simulink model "plant"  (R2016a)
settings: Solver=ode45  StartTime=0.0  StopTime=12  RelTol=1e-3
values from neighbouring files (symbols this model uses):
  A = [1.00008442099 -8.64762700945e-06 -0.00202879786618 -0.0120769175733 -0.00073933561133 1.00039660277 -0.00870367805975 0.00595527209343 -0.00126263380998 0.00387872249587 0.98705447221 -0.0360153373111 ... (16 elements, 4x4)]    [sample.mat]
  B = [-5.50080453987e-08  3.86684801471e-08; 8.77127889262e-08  -5.25096440473e-08; 1.59329018214e-07  1.46974501157e-09; -2.9421226826e-06  9.98312400046e-06]    [sample.mat]
  C = Cbar*C_new    [Params.m]    (also in sample.mat = [0.219326280868  0.071395429974  0.0140743658612  0.00013653)
  m = 3    [Params.m]    (also in Yrates.m = 80)
  p = 5    [Params.m]
  Qu = eye(2)    [Params.m]
  Qy = diag([10000000 10000000 1])    [Params.m]
  Ymeas = Cin(N*p+1:N*p+N)    [Controller.m]    (also in sample.mat = [2 2 200])
undefined symbols (not defined in the file or in its folder): Ref, X0
settings Model: Creator=hp  LastModifiedBy=hp

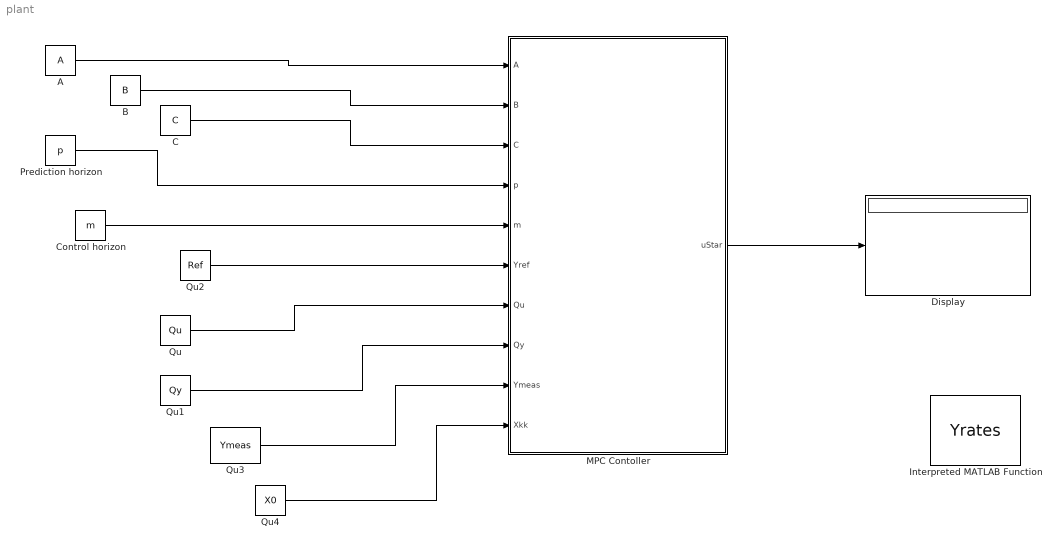
== system plant ==
  A : Constant  Value=A  VectorParams1D=off
  B : Constant  Value=B  VectorParams1D=off
  C : Constant  Value=C  VectorParams1D=off
  Control horizon : Constant  Value=m
  Display : Display
  Interpreted MATLAB Function : MATLABFcn  MATLABFcn=Yrates
  MPC Contoller : MATLAB Function  TreatAsAtomicUnit=on
  Prediction horizon : Constant  Value=p
  Qu : Constant  Value=Qu  VectorParams1D=off
  Qu1 : Constant  Value=Qy  VectorParams1D=off
  Qu2 : Constant  Value=Ref  VectorParams1D=off
  Qu3 : Constant  Value=Ymeas  VectorParams1D=off
  Qu4 : Constant  Value=X0  VectorParams1D=off
  wires:
  MPC Contoller/1(uStar) -> Display/1
  A/1 -> MPC Contoller/1(A)
  B/1 -> MPC Contoller/2(B)
  C/1 -> MPC Contoller/3(C)
  ? -> ?
  Prediction horizon/1 -> MPC Contoller/4(p)
  Control horizon/1 -> MPC Contoller/5(m)
  Qu/1 -> MPC Contoller/7(Qu)
  Qu1/1 -> MPC Contoller/8(Qy)
  Qu2/1 -> MPC Contoller/6(Yref)
  Qu4/1 -> MPC Contoller/10(Xkk)
  Qu3/1 -> MPC Contoller/9(Ymeas)

== matlab function plant/MPC Contoller ==
  data: A input; uStar output size=[2 p] [.. ]; B input; C input; p input [..100]; m input [..p-1]; Yref input; Qu input; Qy input; Ymeas input; Xkk input
function uStar = inputPlanSim(A,B,C, p,m,Yref,Qu,Qy,Ymeas, Xkk)

%{
A,B,C  - State space model matrices
Xkk    - Current estimated state
Yref   - Reference measurement for the prediction horizon size Nxp 
N      - number of measurements
L      - number of inputs
p      - Prediction horizon
m      - control horizon
Qu     - input weights
Qy     - measurement weights
%}

%%
[n, L] = size(B);
[N,~]  = size(C);
H      = zeros(m*L,m*L) ;
f      = zeros(1,m*L) ; 

for i = 1:p
    CABj = CABhoriz(A,B,C,i,m);
    H = H + CABj'*Qy*CABj;
    f = f + Xkk'*(A^i)'*C'*Qy*CABj -Yref(:,i)'*Qy*CABj;
end

% QuBlock = Qu;
% for  b = 1:m-1
%     QuBlock = blkdiag(QuBlock,Qu)
% end
% H = H+QuBlock; 
coder.extrinsic('quadprog');
coder.extrinsic('reshape');
uStar0 = zeros(m*L,1);
uStar0 = quadprog(H,f);
uStar1 = reshape(uStar0,L,[]);
uStar = [uStar1 uStar1(:,end)*ones(1,p-m)];
uStar  = uStar0(1:L);




function CABi=CABhoriz(A,B,C,i,m)

[t,~] = size(C);
[~,s]=size(B);
CABi = zeros(t,s);
if ge(m,i)
    for k=1:i
    CABi = [C*A^(k-1)*B CABi];
    end
 CABi = [ CABi zeros(t,s*(m-i))];
else
    for k=1:m-1
    CABi = [C*A^(k-1)*B CABi];
    end
    At =zeros(t,s);
    for j=1:i-m
       At = At+C*A^j*B; 
    end
    CABi = [CABi At];
end
CABi = CABi(:,1:end-s);
